simulink model "simple_model"  (R2023a)
settings: Solver=FixedStepAuto  StartTime=0.0  StopTime=Tend  FixedStep=Tsim  RelTol=1e-3
values from neighbouring files (symbols this model uses):
  Advanced_clamping_enable = 0    [main.m]
  Back_tracking_enable = 1    [main.m]
  Clamping_enable = 0    [main.m]
  d_ref = 15    [main.m]
  d_step1 = 0.2    [main.m]
  d_step2 = 0.3    [main.m]
  d_step3 = 0.35    [main.m]
  d_step4 = 0.4    [main.m]
  Kb = Ki/Kp    (= 1)    [main.m]
  Ki = wb    (= 62.8318530718)    [main.m]
  Kp = wb    (= 62.8318530718)    [main.m]
  lower_limit = -10    [main.m]
  ref = 0    [main.m]
  start = 0.2    [main.m]
  stop = 1    [main.m]
  upper_limit = 10    [main.m]
settings Model: Creator=tnoguchi  LastModifiedBy=tnoguchi

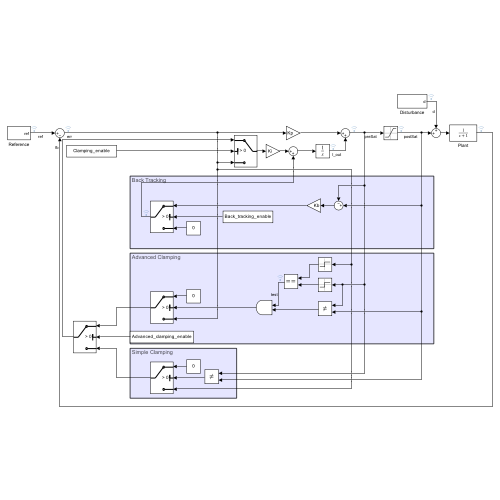
[thumbnail: Simulink's stored preview of the top-level diagram]
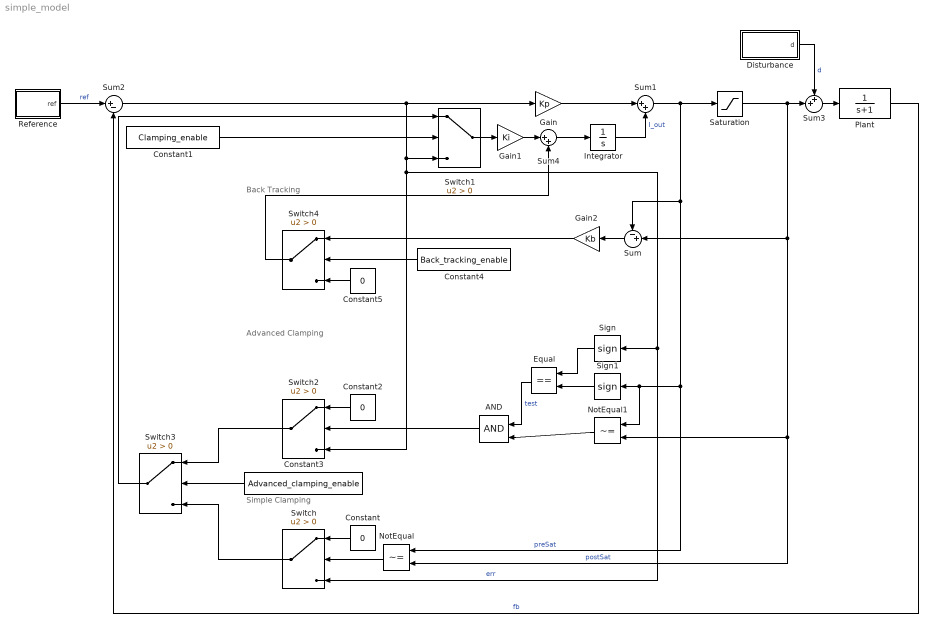
== system simple_model ==
  note: Simple Clamping
  note: Advanced Clamping
  note: Back Tracking
  AND : Logic  IconShape=distinctive  AllPortsSameDT=off  OutDataTypeStr=boolean
  Constant : Constant  Value=0
  Constant1 : Constant  Value=Clamping_enable
  Constant2 : Constant  Value=0
  Constant3 : Constant  Value=Advanced_clamping_enable
  Constant4 : Constant  Value=Back_tracking_enable
  Constant5 : Constant  Value=0
  Disturbance : Subsystem
  Equal : RelationalOperator  Operator===  OutDataTypeStr=boolean  RndMeth=Simplest  InputSameDT=off
  Gain : Gain  Gain=Kp
  Gain1 : Gain  Gain=Ki
  Gain2 : Gain  Gain=Kb
  Integrator : Integrator
  NotEqual : RelationalOperator  Operator=~=  OutDataTypeStr=boolean  RndMeth=Simplest  InputSameDT=off
  NotEqual1 : RelationalOperator  Operator=~=  OutDataTypeStr=boolean  RndMeth=Simplest  InputSameDT=off
  Plant : TransferFcn  Denominator=[1 1]
  Reference : Subsystem
  Saturation : Saturate  UpperLimit=upper_limit  LowerLimit=lower_limit
  Sign : Signum
  Sign1 : Signum
  Sum : Sum  Inputs=-+|
  Sum1 : Sum  Inputs=|++
  Sum2 : Sum  Inputs=|+-
  Sum3 : Sum  Inputs=++|
  Sum4 : Sum  Inputs=|++
  Switch{,1..4} (5 alike) : Switch  Criteria=u2 > Threshold  SaturateOnIntegerOverflow=off  InputSameDT=off
  wires:
  Sum2/1 -> Switch/3, Sign/1, Switch2/3, Switch1/3, Gain/1  "err"
  Plant/1 -> Sum2/2  "fb"
  Sum3/1 -> Plant/1
  Sum1/1 -> NotEqual/1, Sign1/1, NotEqual1/1, Sum/1, Saturation/1  "preSat"
  Saturation/1 -> Sum/2, NotEqual/2, NotEqual1/2, Sum3/2  "postSat"
  NotEqual/1 -> Switch/2
  Constant/1 -> Switch/1
  Reference/1(ref) -> Sum2/1  "ref"
  Disturbance/1(d) -> Sum3/1  "d"
  Constant1/1 -> Switch1/2
  Switch1/1 -> Gain1/1
  NotEqual1/1 -> AND/2
  Sign/1 -> Equal/1
  Sign1/1 -> Equal/2
  Equal/1 -> AND/1  "test"
  AND/1 -> Switch2/2
  Constant2/1 -> Switch2/1
  Switch/1 -> Switch3/3
  Switch2/1 -> Switch3/1
  Constant3/1 -> Switch3/2
  Sum/1 -> Gain2/1
  Gain1/1 -> Sum4/1
  Sum4/1 -> Integrator/1
  Constant4/1 -> Switch4/2
  Gain2/1 -> Switch4/1
  Switch4/1 -> Sum4/2
  Constant5/1 -> Switch4/3
  Switch3/1 -> Switch1/1
  Integrator/1 -> Sum1/2  "I_out"
  Gain/1 -> Sum1/1

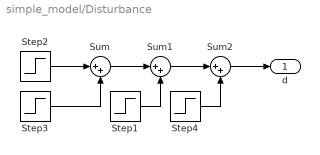
== system simple_model/Disturbance ==
  Step1 : Step  Time=d_step3  After=2*d_ref  SampleTime=0
  Step2 : Step  Time=d_step1  Before=10  After=d_ref  SampleTime=0
  Step3 : Step  Time=d_step2  After=-2*d_ref  SampleTime=0
  Step4 : Step  Time=d_step4  After=-d_ref  SampleTime=0
  Sum : Sum  Inputs=|++
  Sum1 : Sum  Inputs=|++
  Sum2 : Sum  Inputs=|++
  d : Outport
  wires:
  Sum2/1 -> d/1
  Step2/1 -> Sum/1
  Step3/1 -> Sum/2
  Step1/1 -> Sum1/2
  Sum/1 -> Sum1/1
  Sum1/1 -> Sum2/1
  Step4/1 -> Sum2/2

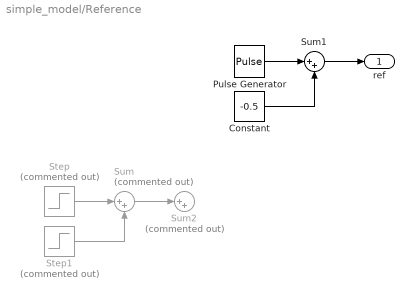
== system simple_model/Reference ==
  Constant : Constant  Value=-0.5
  Pulse Generator : DiscretePulseGenerator  PulseType=Time based  Period=0.05  PulseWidth=50
  Step : Step  Commented=on  Time=start  After=ref  SampleTime=0
  Step1 : Step  Commented=on  Time=stop  After=-5*ref  SampleTime=0
  Sum : Sum  Commented=on  Inputs=|++
  Sum1 : Sum  Inputs=|++
  Sum2 : Sum  Commented=on  Inputs=|++
  ref : Outport
  wires:
  Step/1 -> Sum/1
  Sum/1 -> Sum2/1
  Step1/1 -> Sum/2
  Pulse Generator/1 -> Sum1/1
  Sum1/1 -> ref/1
  Constant/1 -> Sum1/2
